simulink model "SF009A_DutyCycThermProtn"  (R2013b)
settings: Solver=FixedStepDiscrete  SolverMode=SingleTasking  StartTime=0.0  StopTime=1  FixedStep=0.1  RelTol=1e-3
values from neighbouring files (symbols this model uses):
  AbsltTThermLimCnt = DataDict.NTC    [SF009A_DutyCycThermProtn_DataDict.m]
  ARCHGLBPRM_100MILLISEC_SEC_F32 = DataDict.Constant    [SF009A_DutyCycThermProtn_DataDict.m]
  CTRLRANDCUTFLT_CNT_U08 = DataDict.Constant    [SF009A_DutyCycThermProtn_DataDict.m]
  CTRLRTFLT_CNT_U08 = DataDict.Constant    [SF009A_DutyCycThermProtn_DataDict.m]
  CUTFLT_CNT_U08 = DataDict.Constant    [SF009A_DutyCycThermProtn_DataDict.m]
  DITHERMLIM_MOTNWTMTR_F32 = DataDict.Constant    [SF009A_DutyCycThermProtn_DataDict.m]
  DutyCycExcddCnt = DataDict.NTC    [SF009A_DutyCycThermProtn_DataDict.m]
  DutyCycThermProtnAbsltCtrlTTblX = DataDict.Calibration    [SF009A_DutyCycThermProtn_DataDict.m]
  DutyCycThermProtnAbsltCtrlTTqTblY = DataDict.Calibration    [SF009A_DutyCycThermProtn_DataDict.m]
  DutyCycThermProtnAbsltCuTTblX = DataDict.Calibration    [SF009A_DutyCycThermProtn_DataDict.m]
  DutyCycThermProtnAbsltCuTTqTblY = DataDict.Calibration    [SF009A_DutyCycThermProtn_DataDict.m]
  DutyCycThermProtnAbsltMotVelBreakPt = DataDict.Calibration    [SF009A_DutyCycThermProtn_DataDict.m]
  DutyCycThermProtnAbsltTTqSlewHiLim = DataDict.Calibration    [SF009A_DutyCycThermProtn_DataDict.m]
  DutyCycThermProtnAbsltTTqSlewLoLim = DataDict.Calibration    [SF009A_DutyCycThermProtn_DataDict.m]
  DutyCycThermProtnCtrlT = DataDict.Calibration    [SF009A_DutyCycThermProtn_DataDict.m]
  DutyCycThermProtnCtrlTSeln = DataDict.Calibration    [SF009A_DutyCycThermProtn_DataDict.m]
  DutyCycThermProtnDutyCycFildThd = DataDict.Calibration    [SF009A_DutyCycThermProtn_DataDict.m]
  DutyCycThermProtnIgnOffCtrlEna = DataDict.Calibration    [SF009A_DutyCycThermProtn_DataDict.m]
  DutyCycThermProtnIgnOffMsgWaitTi = DataDict.Calibration    [SF009A_DutyCycThermProtn_DataDict.m]
  DutyCycThermProtnLstTblValNonStall = DataDict.Calibration    [SF009A_DutyCycThermProtn_DataDict.m]
  DutyCycThermProtnLstTblValStall = DataDict.Calibration    [SF009A_DutyCycThermProtn_DataDict.m]
  DutyCycThermProtnMotPrTSeln = DataDict.Calibration    [SF009A_DutyCycThermProtn_DataDict.m]
  DutyCycThermProtnMplr1NonStallTblY = DataDict.Calibration    [SF009A_DutyCycThermProtn_DataDict.m]
  DutyCycThermProtnMplr1StallTblY = DataDict.Calibration    [SF009A_DutyCycThermProtn_DataDict.m]
  DutyCycThermProtnMplr2NonStallTblY = DataDict.Calibration    [SF009A_DutyCycThermProtn_DataDict.m]
  DutyCycThermProtnMplr2StallTblY = DataDict.Calibration    [SF009A_DutyCycThermProtn_DataDict.m]
  DutyCycThermProtnMplr3NonStallTblY = DataDict.Calibration    [SF009A_DutyCycThermProtn_DataDict.m]
  DutyCycThermProtnMplr3StallTblY = DataDict.Calibration    [SF009A_DutyCycThermProtn_DataDict.m]
  DutyCycThermProtnMplr4NonStallTblY = DataDict.Calibration    [SF009A_DutyCycThermProtn_DataDict.m]
  DutyCycThermProtnMplr4StallTblY = DataDict.Calibration    [SF009A_DutyCycThermProtn_DataDict.m]
  DutyCycThermProtnMplr5NonStallTblY = DataDict.Calibration    [SF009A_DutyCycThermProtn_DataDict.m]
  DutyCycThermProtnMplr5StallTblY = DataDict.Calibration    [SF009A_DutyCycThermProtn_DataDict.m]
  DutyCycThermProtnMplr6NonStallTblY = DataDict.Calibration    [SF009A_DutyCycThermProtn_DataDict.m]
  DutyCycThermProtnMplr6StallTblY = DataDict.Calibration    [SF009A_DutyCycThermProtn_DataDict.m]
  DutyCycThermProtnMplrTblX = DataDict.Calibration    [SF009A_DutyCycThermProtn_DataDict.m]
  DutyCycThermProtnMplrTSeln = DataDict.Calibration    [SF009A_DutyCycThermProtn_DataDict.m]
  DutyCycThermProtnSlowFilTSeln = DataDict.Calibration    [SF009A_DutyCycThermProtn_DataDict.m]
  DutyCycThermProtnThermLimScaFac = DataDict.Calibration    [SF009A_DutyCycThermProtn_DataDict.m]
  DutyCycThermProtnThermLoadLimTblX = DataDict.Calibration    [SF009A_DutyCycThermProtn_DataDict.m]
  DutyCycThermProtnThermLoadLimTblY = DataDict.Calibration    [SF009A_DutyCycThermProtn_DataDict.m]
  DutyCycThermProtnTqCmdSlewDwn = DataDict.Calibration    [SF009A_DutyCycThermProtn_DataDict.m]
  DutyCycThermProtnTqCmdSlewUp = DataDict.Calibration    [SF009A_DutyCycThermProtn_DataDict.m]
  FILVALMIN_ULS_F32 = DataDict.Constant    [SF009A_DutyCycThermProtn_DataDict.m]
  IGNTIOFFTHD_CNT_F32 = DataDict.Constant    [SF009A_DutyCycThermProtn_DataDict.m]
  NODEBSTEP_CNT_U16 = DataDict.Constant    [SF009A_DutyCycThermProtn_DataDict.m]
  ONEPERC_ULS_F32 = DataDict.Constant    [SF009A_DutyCycThermProtn_DataDict.m]
  TAU3_SEC_F32 = DataDict.Constant    [SF009A_DutyCycThermProtn_DataDict.m]
  TAU4_SEC_F32 = DataDict.Constant    [SF009A_DutyCycThermProtn_DataDict.m]
  TAU5_SEC_F32 = DataDict.Constant    [SF009A_DutyCycThermProtn_DataDict.m]
  TAU6_SEC_F32 = DataDict.Constant    [SF009A_DutyCycThermProtn_DataDict.m]
  THERMLOADLIMTBLIDX_ULS_U08 = DataDict.Constant    [SF009A_DutyCycThermProtn_DataDict.m]
undefined symbols (not defined in the file or in its folder): NtcSts1, NvmGetErrSts1
libraries: FixdToFloat x13, Fil x12, NxtrLim x12, simulink x11, NxtrMath x8, FloatToFixd x6, NxtrMax x6, NxtrMin x3, NxtrAbslt x2, NxtrNvM x1
(part 2 of 7)

== system SF009A_DutyCycThermProtn/DutyCycThermProtn/DutyCycThermProtnInit1/NVM_NOK ==
  note: In the event of NVM failure
      | zero out the whole shadow ram image
  Action Port : ActionPort  ActionType=then
  Constant1 : Constant  RequirementInfo={'linktype_rmi_doors' '0000a52a (/E-STEER Core/SubSystem Specifications/Application Functions/SF009A Thermal Duty Cycle Protection)' '#SF009A_285' 'true' 'REQ: SF009A_285' '' } %GIDa_302cae02_0488_4259_b126_8b47f6fdcb2b  Value=0  OutDataTypeStr=Inherit: Inherit via back propagation
  Constant2 : Constant  RequirementInfo={'linktype_rmi_doors' '0000a52a (/E-STEER Core/SubSystem Specifications/Application Functions/SF009A Thermal Duty Cycle Protection)' '#SF009A_285' 'true' 'REQ: SF009A_285' '' } %GIDa_07daeeb8_67fa_455d_b996_6ae10cb4fd0f  Value=0  OutDataTypeStr=Inherit: Inherit via back propagation
  Constant3 : Constant  RequirementInfo={'linktype_rmi_doors' '0000a52a (/E-STEER Core/SubSystem Specifications/Application Functions/SF009A Thermal Duty Cycle Protection)' '#SF009A_285' 'true' 'REQ: SF009A_285' '' } %GIDa_3e650e9f_6932_4571_90f1_f6987a41f5b5  Value=0  OutDataTypeStr=Inherit: Inherit via back propagation
  Constant4 : Constant  RequirementInfo={'linktype_rmi_doors' '0000a52a (/E-STEER Core/SubSystem Specifications/Application Functions/SF009A Thermal Duty Cycle Protection)' '#SF009A_285' 'true' 'REQ: SF009A_285' '' } %GIDa_9674530a_4135_4c18_b828_962e244c35c9  Value=0  OutDataTypeStr=Inherit: Inherit via back propagation
  CopyRight2 : Subsystem  Description=|  mask(Copyright Information){none=on}
      | Copyright info block.                                               
      |                                                                     
      | Place copyright information at the top of every subsystem in design.
      mask prompts: none "No parameters"
      mask help: Place copyright information at the top of every subsystem in design.
      mask Display:
      | NxtrConf = 'Nexteer Confidential';
      | 
      | sys = bdroot; %handle for the current model ("system")
      | first = get_param(sys,'Created');
      | first = first(end-3:end);  %year is last four digits
      | 
      | last = get_param(sys,'LastModifiedDate');
      | if isempty(last)
      |     last = datestr(now,'yyyy');
      | else
      |     last = last(end-3:end);
      | end
      | 
      | if strcmp(first,last)
      |     fprintf('%s -- Copyright %s Nexteer',NxtrConf,first)
      | else
      |     fprintf('%s -- %s%s- %s Nexteer',NxtrConf,char(169),first,last)
      | end
  Data Store Write2 : DataStoreWrite  RequirementInfo={'linktype_rmi_doors' '0000a52a (/E-STEER Core/SubSystem Specifications/Application Functions/SF009A Thermal Duty Cycle Protection)' '#SF009A_285' 'true' 'REQ: SF009A_285' '' } %GIDa_4ceb1b4c_38bc_44b0_9a64_43020f602cc7  Priority=1  DataStoreName=FilStVal  DataStoreElements=FilStVal.Fil3StVal#FilStVal.Fil4StVal#FilStVal.Fil5StVal#FilStVal.Fil6StVal
  wires:
  Constant1/1 -> Data Store Write2/1
  Constant2/1 -> Data Store Write2/2
  Constant4/1 -> Data Store Write2/4
  Constant3/1 -> Data Store Write2/3

== system SF009A_DutyCycThermProtn/DutyCycThermProtn/DutyCycThermProtnInit1/NVM_Ok ==
  Action Port : ActionPort  ActionType=else
  Constant1 : Constant  Value=0  OutDataTypeStr=Inherit: Inherit via back propagation
  CopyRight2 : Subsystem  Description=|  mask(Copyright Information){none=on}
      | Copyright info block.                                               
      |                                                                     
      | Place copyright information at the top of every subsystem in design.
      mask prompts: none "No parameters"
      mask help: Place copyright information at the top of every subsystem in design.
      mask Display:
      | NxtrConf = 'Nexteer Confidential';
      | 
      | sys = bdroot; %handle for the current model ("system")
      | first = get_param(sys,'Created');
      | first = first(end-3:end);  %year is last four digits
      | 
      | last = get_param(sys,'LastModifiedDate');
      | if isempty(last)
      |     last = datestr(now,'yyyy');
      | else
      |     last = last(end-3:end);
      | end
      | 
      | if strcmp(first,last)
      |     fprintf('%s -- Copyright %s Nexteer',NxtrConf,first)
      | else
      |     fprintf('%s -- %s%s- %s Nexteer',NxtrConf,char(169),first,last)
      | end
  Terminator : Terminator
  wires:
  Constant1/1 -> Terminator/1

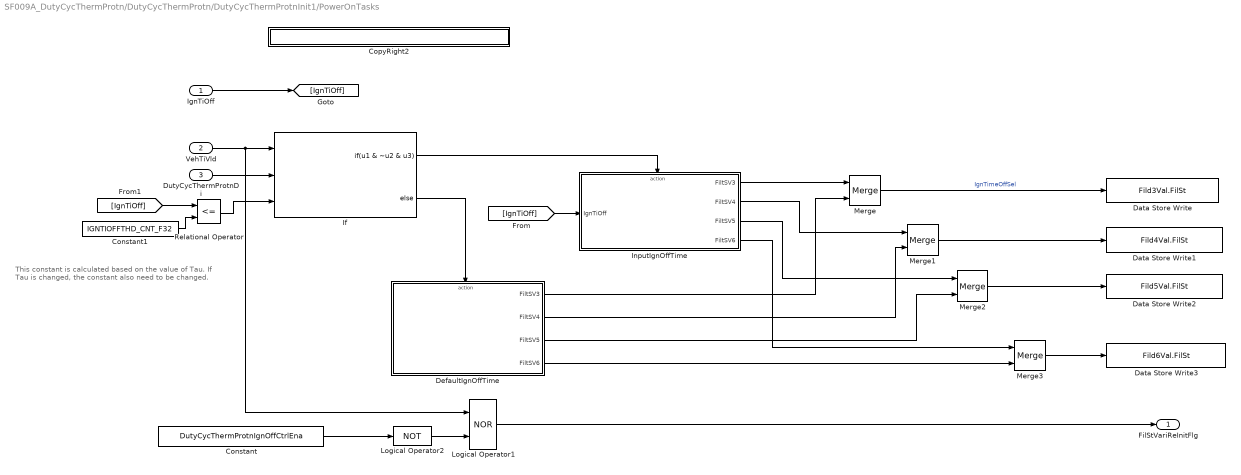
== system SF009A_DutyCycThermProtn/DutyCycThermProtn/DutyCycThermProtnInit1/PowerOnTasks ==
  note: This constant is calculated based on the value of Tau.
      | If Tau is changed, the constant also need to be changed.
  IgnTiOff : Inport
  VehTiVld : Inport  RequirementInfo={'linktype_rmi_doors' '0000a52a (/E-STEER Core/SubSystem Specifications/Application Functions/SF009A Thermal Duty Cycle Protection)' '#SF009A_285' 'true' 'REQ: SF009A_285' '' } %GIDa_9c854dc3_aea9_4b7d_9e72_9615408c52be  Port=2
  DutyCycThermProtnDi : Inport  RequirementInfo={'linktype_rmi_doors' '0000a52a (/E-STEER Core/SubSystem Specifications/Application Functions/SF009A Thermal Duty Cycle Protection)' '#SF009A_285' 'true' 'REQ: SF009A_285' '' } %GIDa_20215133_6a38_4fa5_bfaa_715d5e520197  Port=3
  Constant : Constant  RequirementInfo={'linktype_rmi_doors' '0000a52a (/E-STEER Core/SubSystem Specifications/Application Functions/SF009A Thermal Duty Cycle Protection)' '#SF009A_288' 'true' 'REQ: SF009A_288' '' } %GIDa_d6af1816_8913_46c1_8a5f_e5ae6f6ebd33  Value=DutyCycThermProtnIgnOffCtrlEna
  Constant1 : Constant  RequirementInfo={'linktype_rmi_doors' '0000a52a (/E-STEER Core/SubSystem Specifications/Application Functions/SF009A Thermal Duty Cycle Protection)' '#SF009A_285' 'true' 'REQ: SF009A_285' '' } %GIDa_da13bd96_169e_43ad_9aad_13a1d233c3db  Value=IGNTIOFFTHD_CNT_F32
  CopyRight2 : Subsystem  Description=|  mask(Copyright Information){none=on}
      | Copyright info block.                                               
      |                                                                     
      | Place copyright information at the top of every subsystem in design.
      mask prompts: none "No parameters"
      mask help: Place copyright information at the top of every subsystem in design.
      mask Display:
      | NxtrConf = 'Nexteer Confidential';
      | 
      | sys = bdroot; %handle for the current model ("system")
      | first = get_param(sys,'Created');
      | first = first(end-3:end);  %year is last four digits
      | 
      | last = get_param(sys,'LastModifiedDate');
      | if isempty(last)
      |     last = datestr(now,'yyyy');
      | else
      |     last = last(end-3:end);
      | end
      | 
      | if strcmp(first,last)
      |     fprintf('%s -- Copyright %s Nexteer',NxtrConf,first)
      | else
      |     fprintf('%s -- %s%s- %s Nexteer',NxtrConf,char(169),first,last)
      | end
  Data Store Write : DataStoreWrite  DataStoreName=Fild3Val  DataStoreElements=Fild3Val.FilSt
  Data Store Write1 : DataStoreWrite  DataStoreName=Fild4Val  DataStoreElements=Fild4Val.FilSt
  Data Store Write2 : DataStoreWrite  DataStoreName=Fild5Val  DataStoreElements=Fild5Val.FilSt
  Data Store Write3 : DataStoreWrite  DataStoreName=Fild6Val  DataStoreElements=Fild6Val.FilSt
  DefaultIgnOffTime : Subsystem  RequirementInfo={} %GIDa_e2463be5_64da_4144_9cc6_dd109eab91a1  TreatAsAtomicUnit=on
  If : If  RequirementInfo={'linktype_rmi_doors' '0000a52a (/E-STEER Core/SubSystem Specifications/Application Functions/SF009A Thermal Duty Cycle Protection)' '#SF009A_285' 'true' 'REQ: SF009A_285' '' } %GIDa_3e38b5b9_0c5d_47ab_89b1_64e918870a53  NumInputs=3  IfExpression=u1 & ~u2 & u3
  InputIgnOffTime : Subsystem  RequirementInfo={} %GIDa_43daa1c3_65fe_4cdd_94a1_b7322396a1ac  TreatAsAtomicUnit=on
  Logical Operator1 : Logic  RequirementInfo={'linktype_rmi_doors' '0000a52a (/E-STEER Core/SubSystem Specifications/Application Functions/SF009A Thermal Duty Cycle Protection)' '#SF009A_280' 'true' 'REQ: SF009A_280' '' } %GIDa_edbebf0e_bcf8_4967_a510_970fba2b2e0b  Operator=NOR  AllPortsSameDT=off  OutDataTypeStr=boolean
  Logical Operator2 : Logic  RequirementInfo={'linktype_rmi_doors' '0000a52a (/E-STEER Core/SubSystem Specifications/Application Functions/SF009A Thermal Duty Cycle Protection)' '#SF009A_280' 'true' 'REQ: SF009A_280' '' } %GIDa_f304b822_166f_4701_8c8b_94ad225b72e6  Operator=NOT  AllPortsSameDT=off  OutDataTypeStr=boolean
  Merge : Merge  RequirementInfo={} %GIDa_1e03ac42_f159_46b0_a200_7b6c92e2721c
  Merge1 : Merge  RequirementInfo={} %GIDa_32e162cf_165c_4a40_9f13_19e0e5e6e227
  Merge2 : Merge  RequirementInfo={} %GIDa_493fd6f9_28e3_4a2f_8c16_2836a030636e
  Merge3 : Merge  RequirementInfo={} %GIDa_b95078aa_c4af_4ddb_8213_bc830cf1fee0
  Relational Operator : RelationalOperator  RequirementInfo={'linktype_rmi_doors' '0000a52a (/E-STEER Core/SubSystem Specifications/Application Functions/SF009A Thermal Duty Cycle Protection)' '#SF009A_285' 'true' 'REQ: SF009A_285' '' } %GIDa_8a99ca10_b364_4588_b658_259f4470d472  Operator=<=  OutDataTypeStr=boolean
  FilStVariReInitFlg : Outport
  wires:
  Logical Operator1/1 -> FilStVariReInitFlg/1
  Constant/1 -> Logical Operator2/1
  VehTiVld/1 -> If/1, Logical Operator1/1
  Logical Operator2/1 -> Logical Operator1/2
  DutyCycThermProtnDi/1 -> If/2
  [IgnTiOff] -> InputIgnOffTime/1(IgnTiOff)
  If/1 -> InputIgnOffTime/Action
  InputIgnOffTime/1(FiltSV3) -> Merge/1
  DefaultIgnOffTime/1(FiltSV3) -> Merge/2
  If/2 -> DefaultIgnOffTime/Action
  IgnTiOff/1 -> [IgnTiOff]
  [IgnTiOff] -> Relational Operator/1
  Constant1/1 -> Relational Operator/2
  Relational Operator/1 -> If/3
  DefaultIgnOffTime/2(FiltSV4) -> Merge1/2
  InputIgnOffTime/2(FiltSV4) -> Merge1/1
  InputIgnOffTime/3(FiltSV5) -> Merge2/1
  DefaultIgnOffTime/3(FiltSV5) -> Merge2/2
  InputIgnOffTime/4(FiltSV6) -> Merge3/1
  DefaultIgnOffTime/4(FiltSV6) -> Merge3/2
  Merge3/1 -> Data Store Write3/1
  Merge2/1 -> Data Store Write2/1
  Merge1/1 -> Data Store Write1/1
  Merge/1 -> Data Store Write/1  "IgnTimeOffSel"

== system SF009A_DutyCycThermProtn/DutyCycThermProtn/DutyCycThermProtnInit1/SetInitialValueOfAbsTempLimitSlew ==
  note: This subsystem sets the initial value of the "AbsltTLimSlewStVari"
      | which is used as state variable of rate limiter block in Per1 subsystem.
  Constant2 : Constant  Value=0
  Copyright1 : Subsystem  Description=|  RequirementInfo={} %GIDa_1a6fa9aa_8716_46b8_8e70_044847d882f9  mask(Copyright Information){none=on}
      | Copyright info block.                                               
      |                                                                     
      | Place copyright information at the top of every subsystem in design.
      mask prompts: none "No parameters"
      mask help: Place copyright information at the top of every subsystem in design.
      mask Display:
      | NxtrConf = 'Nexteer Confidential';
      | 
      | sys = bdroot; %handle for the current model ("system")
      | first = get_param(sys,'Created');
      | if(isempty(first))
      |     first = datestr(now,'yyyy');
      | else
      |     first = first(end-3:end);  %year is last four digits
      | end
      | 
      | last = get_param(sys,'LastModifiedDate');
      | if isempty(last)
      |     last = datestr(now,'yyyy');
      | else
      |     last = last(end-3:end);
      | end
      | 
      | if strcmp(first,last)
      |     fprintf('%s\nCopyright  %s Nexteer',NxtrConf,first);
      | else
      |     fprintf('%s\n%s%s-%s Nexteer',NxtrConf,char(169),first,last);
      | end
  Data Store Write : DataStoreWrite  DataStoreName=AbsltTLimSlewStVari
  FixdToFloat_f32_u16 : FixdToFloat/FixdToFloat_f32_u16  Param1=7
  Selector2 : Selector  IndexMode=Zero-based  InputPortWidth=4  IndexOptions=Index vector (port)  Indices=[1 3]  OutputSizes=1
  const2 : Constant  Value=DutyCycThermProtnAbsltCtrlTTqTblY
  wires:
  Selector2/1 -> FixdToFloat_f32_u16/1
  const2/1 -> Selector2/1
  Constant2/1 -> Selector2/2
  FixdToFloat_f32_u16/1 -> Data Store Write/1

== system SF009A_DutyCycThermProtn/DutyCycThermProtn/DutyCycThermProtnInit1/SetInitialValueOfLstTblValRateLimrStVari ==
  note: Last value of the table "DutyCycThermProtnThermLoadLimTblY" is selected and assigned to "LstTblValRateLimrStVari".
  note: This subsystem sets the initial value of the "LstTblValRateLimrStVari"
      | which is used as state variable of rate limiter block in Per1 subsystem.
  Add : Sum  Inputs=+-
  Constant1 : Constant  OutDataTypeStr=uint8
  Constant3 : Constant  Value=THERMLOADLIMTBLIDX_ULS_U08
  Copyright1 : Subsystem  Description=|  RequirementInfo={} %GIDa_56626e63_5a4b_4b9f_b0a2_c0ad22b87c06  mask(Copyright Information){none=on}
      | Copyright info block.                                               
      |                                                                     
      | Place copyright information at the top of every subsystem in design.
      mask prompts: none "No parameters"
      mask help: Place copyright information at the top of every subsystem in design.
      mask Display:
      | NxtrConf = 'Nexteer Confidential';
      | 
      | sys = bdroot; %handle for the current model ("system")
      | first = get_param(sys,'Created');
      | if(isempty(first))
      |     first = datestr(now,'yyyy');
      | else
      |     first = first(end-3:end);  %year is last four digits
      | end
      | 
      | last = get_param(sys,'LastModifiedDate');
      | if isempty(last)
      |     last = datestr(now,'yyyy');
      | else
      |     last = last(end-3:end);
      | end
      | 
      | if strcmp(first,last)
      |     fprintf('%s\nCopyright  %s Nexteer',NxtrConf,first);
      | else
      |     fprintf('%s\n%s%s-%s Nexteer',NxtrConf,char(169),first,last);
      | end
  Data Store Write : DataStoreWrite  DataStoreName=LstTblValRateLimrStVari
  FixdToFloat_f32_u16 : FixdToFloat/FixdToFloat_f32_u16  Param1=7
  Selector2 : Selector  IndexMode=Zero-based  InputPortWidth=8  IndexOptions=Index vector (port)  Indices=[1 3]  OutputSizes=1
  const1 : Constant  Value=DutyCycThermProtnThermLoadLimTblY
  wires:
  const1/1 -> Selector2/1
  Constant3/1 -> Add/1
  FixdToFloat_f32_u16/1 -> Data Store Write/1
  Selector2/1 -> FixdToFloat_f32_u16/1
  Constant1/1 -> Add/2
  Add/1 -> Selector2/2

== system SF009A_DutyCycThermProtn/DutyCycThermProtn/DutyCycThermProtnPer1/CopyRight2 ==

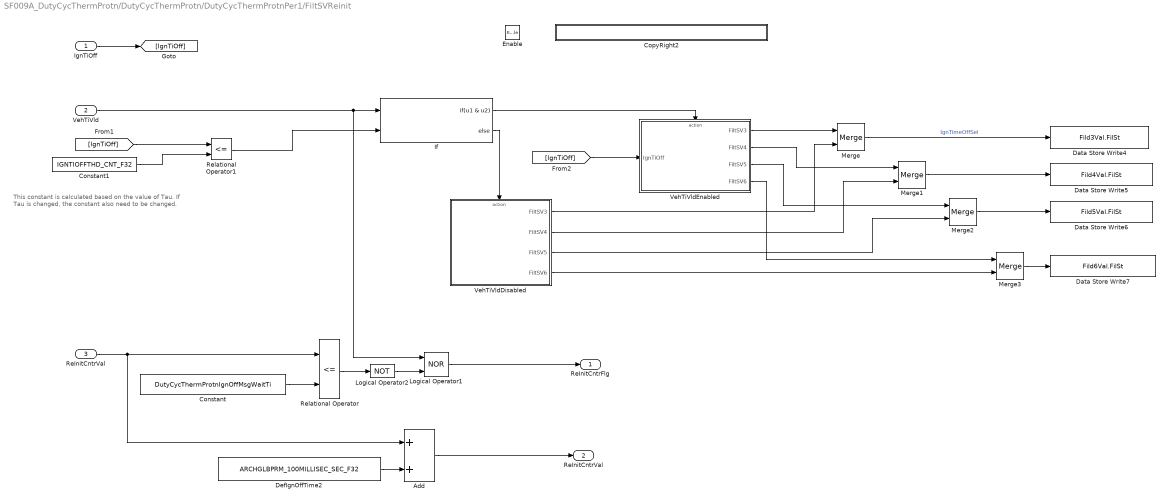
== system SF009A_DutyCycThermProtn/DutyCycThermProtn/DutyCycThermProtnPer1/FiltSVReinit ==
  note: This constant is calculated based on the value of Tau.
      | If Tau is changed, the constant also need to be changed.
  "IgnTiOff " : Inport
  VehTiVld : Inport  RequirementInfo={'linktype_rmi_doors' '0000a52a (/E-STEER Core/SubSystem Specifications/Application Functions/SF009A Thermal Duty Cycle Protection)' '#SF009A_285' 'true' 'REQ: SF009A_285' '' } %GIDa_f2cd1e6f_4c09_4c7d_bb23_8c8b610d12b5  Port=2
  "ReInitCntrVal " : Inport  Port=3
  Enable : EnablePort
  Add : Sum  RequirementInfo={'linktype_rmi_doors' '0000a52a (/E-STEER Core/SubSystem Specifications/Application Functions/SF009A Thermal Duty Cycle Protection)' '#SF009A_280' 'true' 'REQ: SF009A_280' '' } %GIDa_580a5325_9da3_4dde_9987_9ed8cd772d3d
  Constant : Constant  RequirementInfo={'linktype_rmi_doors' '0000a52a (/E-STEER Core/SubSystem Specifications/Application Functions/SF009A Thermal Duty Cycle Protection)' '#SF009A_280' 'true' 'REQ: SF009A_280' '' } %GIDa_c76ac90e_c62d_4456_ae2a_df3b21a2a4e0  Value=DutyCycThermProtnIgnOffMsgWaitTi
  Constant1 : Constant  RequirementInfo={'linktype_rmi_doors' '0000a52a (/E-STEER Core/SubSystem Specifications/Application Functions/SF009A Thermal Duty Cycle Protection)' '#SF009A_285' 'true' 'REQ: SF009A_285' '' } %GIDa_846e87e9_58bc_4580_b93b_af0c098bc72a  Value=IGNTIOFFTHD_CNT_F32
  CopyRight2 : Subsystem  Description=|  mask(Copyright Information){none=on}
      | Copyright info block.                                               
      |                                                                     
      | Place copyright information at the top of every subsystem in design.
      mask prompts: none "No parameters"
      mask help: Place copyright information at the top of every subsystem in design.
      mask Display:
      | NxtrConf = 'Nexteer Confidential';
      | 
      | sys = bdroot; %handle for the current model ("system")
      | first = get_param(sys,'Created');
      | first = first(end-3:end);  %year is last four digits
      | 
      | last = get_param(sys,'LastModifiedDate');
      | if isempty(last)
      |     last = datestr(now,'yyyy');
      | else
      |     last = last(end-3:end);
      | end
      | 
      | if strcmp(first,last)
      |     fprintf('%s -- Copyright %s Nexteer',NxtrConf,first)
      | else
      |     fprintf('%s -- %s%s- %s Nexteer',NxtrConf,char(169),first,last)
      | end
  Data Store Write4 : DataStoreWrite  DataStoreName=Fild3Val  DataStoreElements=Fild3Val.FilSt
  Data Store Write5 : DataStoreWrite  DataStoreName=Fild4Val  DataStoreElements=Fild4Val.FilSt
  Data Store Write6 : DataStoreWrite  DataStoreName=Fild5Val  DataStoreElements=Fild5Val.FilSt
  Data Store Write7 : DataStoreWrite  DataStoreName=Fild6Val  DataStoreElements=Fild6Val.FilSt
  DefIgnOffTime2 : Constant  RequirementInfo={'linktype_rmi_doors' '0000a52a (/E-STEER Core/SubSystem Specifications/Application Functions/SF009A Thermal Duty Cycle Protection)' '#SF009A_280' 'true' 'REQ: SF009A_280' '' } %GIDa_5fa57ba4_c528_4fb6_a79f_ab3413b38764  Value=ARCHGLBPRM_100MILLISEC_SEC_F32
  If : If  RequirementInfo={'linktype_rmi_doors' '0000a52a (/E-STEER Core/SubSystem Specifications/Application Functions/SF009A Thermal Duty Cycle Protection)' '#SF009A_285' 'true' 'REQ: SF009A_285' '' } %GIDa_6e003379_c095_4539_a389_1aacbace0d02  NumInputs=2  IfExpression=u1 & u2
  Logical Operator1 : Logic  RequirementInfo={'linktype_rmi_doors' '0000a52a (/E-STEER Core/SubSystem Specifications/Application Functions/SF009A Thermal Duty Cycle Protection)' '#SF009A_280' 'true' 'REQ: SF009A_280' '' } %GIDa_284f8ad3_0460_4306_9723_53fb8582929e  Operator=NOR  AllPortsSameDT=off  OutDataTypeStr=boolean
  Logical Operator2 : Logic  RequirementInfo={'linktype_rmi_doors' '0000a52a (/E-STEER Core/SubSystem Specifications/Application Functions/SF009A Thermal Duty Cycle Protection)' '#SF009A_280' 'true' 'REQ: SF009A_280' '' } %GIDa_ec00b3f8_66ee_40a8_b7f7_19a445abbf83  Operator=NOT  AllPortsSameDT=off  OutDataTypeStr=boolean
  Merge : Merge  RequirementInfo={} %GIDa_fbbdd3d2_97f2_48a8_a46c_7182b36b6720
  Merge1 : Merge  RequirementInfo={} %GIDa_e9f01da1_ad1a_48a2_b9b1_8b84a4874e09
  Merge2 : Merge  RequirementInfo={} %GIDa_ac698b32_b42d_493c_a1a9_4f85f963d138
  Merge3 : Merge  RequirementInfo={} %GIDa_ea067629_621b_4d75_9cda_f744346af075
  Relational Operator : RelationalOperator  RequirementInfo={'linktype_rmi_doors' '0000a52a (/E-STEER Core/SubSystem Specifications/Application Functions/SF009A Thermal Duty Cycle Protection)' '#SF009A_280' 'true' 'REQ: SF009A_280' '' } %GIDa_3f2901e1_9a76_40d7_87e1_0b54f413400c  Operator=<=  OutDataTypeStr=boolean
  Relational Operator1 : RelationalOperator  RequirementInfo={'linktype_rmi_doors' '0000a52a (/E-STEER Core/SubSystem Specifications/Application Functions/SF009A Thermal Duty Cycle Protection)' '#SF009A_285' 'true' 'REQ: SF009A_285' '' } %GIDa_8f6b1d28_5bfc_46ec_8742_0f7436e122d1  Operator=<=  OutDataTypeStr=boolean
  VehTiVldDisabled : Subsystem  RequirementInfo={} %GIDa_324970fa_b22f_49af_a8a8_20d743678a1e  TreatAsAtomicUnit=on
  VehTiVldEnabled : Subsystem  RequirementInfo={} %GIDa_999d4a90_5417_41b8_9c74_fb77c55787e8  TreatAsAtomicUnit=on
  ReInitCntrFlg : Outport
  ReInitCntrVal : Outport  Port=2
  wires:
  VehTiVld/1 -> Logical Operator1/1, If/1
  Relational Operator/1 -> Logical Operator2/1
  Logical Operator1/1 -> ReInitCntrFlg/1
  Constant/1 -> Relational Operator/2
  "ReInitCntrVal "/1 -> Relational Operator/1, Add/1
  DefIgnOffTime2/1 -> Add/2
  Add/1 -> ReInitCntrVal/1
  Logical Operator2/1 -> Logical Operator1/2
  "IgnTiOff "/1 -> [IgnTiOff]
  If/1 -> VehTiVldEnabled/Action
  If/2 -> VehTiVldDisabled/Action
  VehTiVldEnabled/1(FiltSV3) -> Merge/1
  VehTiVldDisabled/1(FiltSV3) -> Merge/2
  VehTiVldEnabled/2(FiltSV4) -> Merge1/1
  VehTiVldDisabled/2(FiltSV4) -> Merge1/2
  VehTiVldEnabled/3(FiltSV5) -> Merge2/1
  VehTiVldDisabled/3(FiltSV5) -> Merge2/2
  VehTiVldDisabled/4(FiltSV6) -> Merge3/2
  VehTiVldEnabled/4(FiltSV6) -> Merge3/1
  Merge/1 -> Data Store Write4/1  "IgnTimeOffSel"
  Merge1/1 -> Data Store Write5/1
  Merge2/1 -> Data Store Write6/1
  Merge3/1 -> Data Store Write7/1
  Constant1/1 -> Relational Operator1/2
  [IgnTiOff] -> Relational Operator1/1
  Relational Operator1/1 -> If/2
  [IgnTiOff] -> VehTiVldEnabled/1(IgnTiOff)

== system SF009A_DutyCycThermProtn/DutyCycThermProtn/DutyCycThermProtnPer1/LoadLimiting ==
  MotCurrPeakEstimd : Inport
  MotCurrPeakEstimdFild : Inport  Port=2
  MotVelCrf : Inport  Port=3
  Mult12Temp : Inport  Port=4
  Mult36Temp : Inport  Port=5
  SlcTemp : Inport  Port=6
  DutyCycThermProtnDi : Inport  Port=7
  CopyRight2 : Subsystem  Description=|  mask(Copyright Information){none=on}
      | Copyright info block.                                               
      |                                                                     
      | Place copyright information at the top of every subsystem in design.
      mask prompts: none "No parameters"
      mask help: Place copyright information at the top of every subsystem in design.
      mask Display:
      | NxtrConf = 'Nexteer Confidential';
      | 
      | sys = bdroot; %handle for the current model ("system")
      | first = get_param(sys,'Created');
      | first = first(end-3:end);  %year is last four digits
      | 
      | last = get_param(sys,'LastModifiedDate');
      | if isempty(last)
      |     last = datestr(now,'yyyy');
      | else
      |     last = last(end-3:end);
      | end
      | 
      | if strcmp(first,last)
      |     fprintf('%s -- Copyright %s Nexteer',NxtrConf,first)
      | else
      |     fprintf('%s -- %s%s- %s Nexteer',NxtrConf,char(169),first,last)
      | end
  FilterPercMax : Subsystem  RequirementInfo={'linktype_rmi_doors' '0000a52a (/E-STEER Core/SubSystem Specifications/Application Functions/SF009A Thermal Duty Cycle Protection)' '#SF009A_117' 'true' 'REQ: SF009A_117' '' ; 'linktype_rmi_doors' '0000a52a (/E-STEER Core/SubSystem Specifications/Application Functions/SF009A Thermal Duty Cycle Protection)' '#SF009A_164' 'true' 'REQ: SF009A_164' '' ; 'linktype_rmi_doors' '0000a52a (/E-STEER Core/SubSystem Specifications/Application Functions/SF009A Thermal Duty Cycle Protection)' '#SF009A_167' 'true' 'REQ: SF009A_167' '' } %GIDa_3ed6a9be_a9c0_4455_85d8_2437f2a07ac3
  Multiplier : Subsystem  RequirementInfo={'linktype_rmi_doors' '0000a52a (/E-STEER Core/SubSystem Specifications/Application Functions/SF009A Thermal Duty Cycle Protection)' '#SF009A_155' 'true' 'REQ: SF009A_155' '' } %GIDa_6617263c_fa09_4775_af12_9c4ea5a67b95
  PowerOffTasks : Subsystem  RequirementInfo={} %GIDa_972c5a1a_4225_44ec_a602_2278b884c0a1
  ThermalLoadLimit : Subsystem  RequirementInfo={} %GIDa_b466cb19_a628_4d86_8b51_80f6cd1be6a8
  ThermLimSlowFilMax : Outport
  DutyCycThermProtnMaxOutp : Outport  Port=2
  ThermalLoadLmt : Outport  Port=3
  wires:
  Mult12Temp/1 -> Multiplier/1(Mult12Temp)
  Mult36Temp/1 -> Multiplier/2(Mult36Temp)
  MotCurrPeakEstimd/1 -> FilterPercMax/7(MotCurrPeakEstimd)
  MotCurrPeakEstimdFild/1 -> FilterPercMax/8(MotCurrPeakEstimdFild)
  ThermalLoadLimit/1(ThermalLoadLmt) -> ThermalLoadLmt/1
  FilterPercMax/1(MaxOut) -> ThermalLoadLimit/3(MaxOut), DutyCycThermProtnMaxOutp/1
  SlcTemp/1 -> ThermalLoadLimit/2(SlcTemp)
  FilterPercMax/2(ThermLimSlowFilMax) -> ThermLimSlowFilMax/1
  Multiplier/1(Mult1) -> FilterPercMax/1(Mult1)
  Multiplier/2(Mult2) -> FilterPercMax/2(Mult2)
  Multiplier/3(Mult3) -> FilterPercMax/3(Mult3)
  Multiplier/4(Mult4) -> FilterPercMax/4(Mult4)
  Multiplier/5(Mult5) -> FilterPercMax/5(Mult5)
  Multiplier/6(Mult6) -> FilterPercMax/6(Mult6)
  MotVelCrf/1 -> Multiplier/3(MotVelCrf), [MtrVel]
  [MtrVel] -> ThermalLoadLimit/1(MotVelCrf)
  DutyCycThermProtnDi/1 -> FilterPercMax/9(DutyCycThermProtnDi)

== system SF009A_DutyCycThermProtn/DutyCycThermProtn/DutyCycThermProtnPer1/ServiceDefeatFiltSVReinit ==
  Enable : EnablePort
  CopyRight2 : Subsystem  Description=|  mask(Copyright Information){none=on}
      | Copyright info block.                                               
      |                                                                     
      | Place copyright information at the top of every subsystem in design.
      mask prompts: none "No parameters"
      mask help: Place copyright information at the top of every subsystem in design.
      mask Display:
      | NxtrConf = 'Nexteer Confidential';
      | 
      | sys = bdroot; %handle for the current model ("system")
      | first = get_param(sys,'Created');
      | first = first(end-3:end);  %year is last four digits
      | 
      | last = get_param(sys,'LastModifiedDate');
      | if isempty(last)
      |     last = datestr(now,'yyyy');
      | else
      |     last = last(end-3:end);
      | end
      | 
      | if strcmp(first,last)
      |     fprintf('%s -- Copyright %s Nexteer',NxtrConf,first)
      | else
      |     fprintf('%s -- %s%s- %s Nexteer',NxtrConf,char(169),first,last)
      | end
  Data Store Write : DataStoreWrite  DataStoreName=Fild3Val  DataStoreElements=Fild3Val.FilSt
  Data Store Write1 : DataStoreWrite  DataStoreName=Fild4Val  DataStoreElements=Fild4Val.FilSt
  Data Store Write2 : DataStoreWrite  DataStoreName=Fild5Val  DataStoreElements=Fild5Val.FilSt
  Data Store Write3 : DataStoreWrite  DataStoreName=Fild6Val  DataStoreElements=Fild6Val.FilSt
  DefIgnOffTime1 : Constant  Value=FILVALMIN_ULS_F32
  wires:
  DefIgnOffTime1/1 -> Data Store Write2/1, Data Store Write3/1, Data Store Write1/1, Data Store Write/1

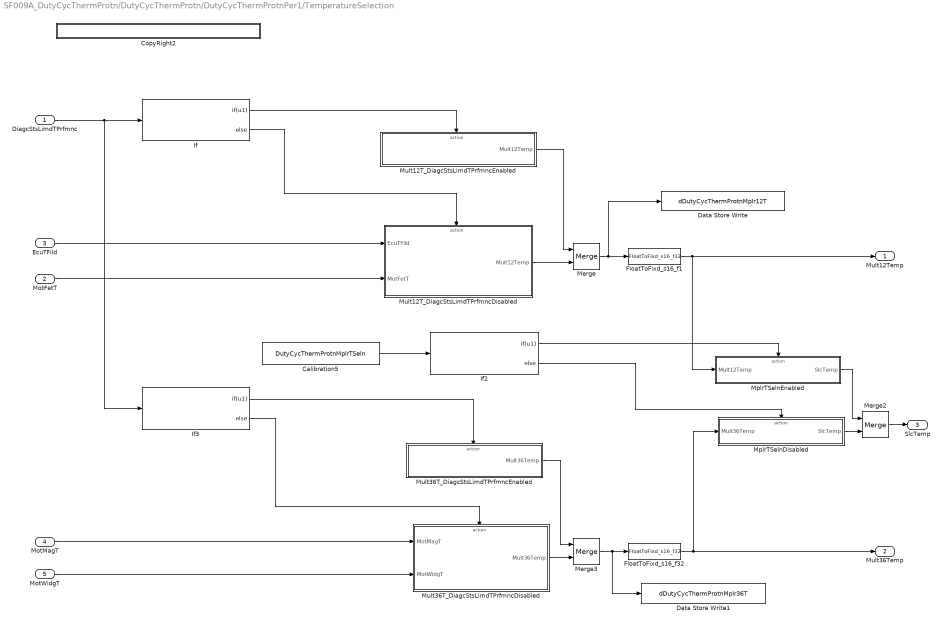
== system SF009A_DutyCycThermProtn/DutyCycThermProtn/DutyCycThermProtnPer1/TemperatureSelection ==
  DiagcStsLimdTPrfmnc : Inport
  MotFetT : Inport  Port=2
  EcuTFild : Inport  Port=3
  MotMagT : Inport  Port=4
  MotWidgT : Inport  Port=5
  Calibration5 : Constant  RequirementInfo={'linktype_rmi_doors' '0000a52a (/E-STEER Core/SubSystem Specifications/Application Functions/SF009A Thermal Duty Cycle Protection)' '#SF009A_114' 'true' 'REQ: SF009A_114' '' } %GIDa_8e23093e_27f7_4ecb_a00e_278a1ac33baa  Value=DutyCycThermProtnMplrTSeln
  CopyRight2 : Subsystem  Description=|  mask(Copyright Information){none=on}
      | Copyright info block.                                               
      |                                                                     
      | Place copyright information at the top of every subsystem in design.
      mask prompts: none "No parameters"
      mask help: Place copyright information at the top of every subsystem in design.
      mask Display:
      | NxtrConf = 'Nexteer Confidential';
      | 
      | sys = bdroot; %handle for the current model ("system")
      | first = get_param(sys,'Created');
      | first = first(end-3:end);  %year is last four digits
      | 
      | last = get_param(sys,'LastModifiedDate');
      | if isempty(last)
      |     last = datestr(now,'yyyy');
      | else
      |     last = last(end-3:end);
      | end
      | 
      | if strcmp(first,last)
      |     fprintf('%s -- Copyright %s Nexteer',NxtrConf,first)
      | else
      |     fprintf('%s -- %s%s- %s Nexteer',NxtrConf,char(169),first,last)
      | end
  Data Store Write : DataStoreWrite  DataStoreName=dDutyCycThermProtnMplr12T
  Data Store Write1 : DataStoreWrite  DataStoreName=dDutyCycThermProtnMplr36T
  FloatToFixd_s16_f1 : FloatToFixd/FloatToFixd_s16_f32  Param1=0
  FloatToFixd_s16_f32 : FloatToFixd/FloatToFixd_s16_f32  Param1=0
  If : If  RequirementInfo={'linktype_rmi_doors' '0000a52a (/E-STEER Core/SubSystem Specifications/Application Functions/SF009A Thermal Duty Cycle Protection)' '#SF009A_184' 'true' 'REQ: SF009A_184' '' } %GIDa_ca8a8c74_c39c_4f29_8ea9_80465840cae0  IfExpression=u1
  If2 : If  RequirementInfo={'linktype_rmi_doors' '0000a52a (/E-STEER Core/SubSystem Specifications/Application Functions/SF009A Thermal Duty Cycle Protection)' '#SF009A_114' 'true' 'REQ: SF009A_114' '' } %GIDa_9b47838e_1e46_4d53_a4ac_947f8f2c2970  IfExpression=u1
  If3 : If  RequirementInfo={'linktype_rmi_doors' '0000a52a (/E-STEER Core/SubSystem Specifications/Application Functions/SF009A Thermal Duty Cycle Protection)' '#SF009A_188' 'true' 'REQ: SF009A_188' '' } %GIDa_e0f30479_aede_45c0_8abe_02078f308a8d  IfExpression=u1
  Merge : Merge  RequirementInfo={'linktype_rmi_doors' '0000a52a (/E-STEER Core/SubSystem Specifications/Application Functions/SF009A Thermal Duty Cycle Protection)' '#SF009A_184' 'true' 'REQ: SF009A_184' '' } %GIDa_1e2f67ed_7672_410c_a92f_4fda9fc6bd3d
  Merge2 : Merge  RequirementInfo={'linktype_rmi_doors' '0000a52a (/E-STEER Core/SubSystem Specifications/Application Functions/SF009A Thermal Duty Cycle Protection)' '#SF009A_114' 'true' 'REQ: SF009A_114' '' } %GIDa_8d348bab_bea0_492a_9b59_59bbd08be9d5
  Merge3 : Merge  RequirementInfo={'linktype_rmi_doors' '0000a52a (/E-STEER Core/SubSystem Specifications/Application Functions/SF009A Thermal Duty Cycle Protection)' '#SF009A_188' 'true' 'REQ: SF009A_188' '' } %GIDa_5df8e3ee_3e2f_4cf5_813e_794d96b1672c
  MplrTSelnDisabled : Subsystem  RequirementInfo={'linktype_rmi_doors' '0000a52a (/E-STEER Core/SubSystem Specifications/Application Functions/SF009A Thermal Duty Cycle Protection)' '#SF009A_114' 'true' 'REQ: SF009A_114' '' } %GIDa_152d6577_ddba_4ed6_964d_7fee3b02f844  TreatAsAtomicUnit=on
  MplrTSelnEnabled : Subsystem  RequirementInfo={'linktype_rmi_doors' '0000a52a (/E-STEER Core/SubSystem Specifications/Application Functions/SF009A Thermal Duty Cycle Protection)' '#SF009A_114' 'true' 'REQ: SF009A_114' '' } %GIDa_cce2fbea_6a9c_432f_a513_853a7592208d  TreatAsAtomicUnit=on
  Mult12T_DiagcStsLimdTPrfmncDisabled : Subsystem  RequirementInfo={'linktype_rmi_doors' '0000a52a (/E-STEER Core/SubSystem Specifications/Application Functions/SF009A Thermal Duty Cycle Protection)' '#SF009A_184' 'true' 'REQ: SF009A_184' '' ; 'linktype_rmi_doors' '0000a52a (/E-STEER Core/SubSystem Specifications/Application Functions/SF009A Thermal Duty Cycle Protection)' '#SF009A_113' 'true' 'REQ: SF009A_113' '' } %GIDa_200d0c66_213e_4297_a369_dd30af9723bb  TreatAsAtomicUnit=on
  Mult12T_DiagcStsLimdTPrfmncEnabled : Subsystem  RequirementInfo={'linktype_rmi_doors' '0000a52a (/E-STEER Core/SubSystem Specifications/Application Functions/SF009A Thermal Duty Cycle Protection)' '#SF009A_184' 'true' 'REQ: SF009A_184' '' } %GIDa_a9e4a746_b9d3_4349_8af5_fb55dffcf03f  TreatAsAtomicUnit=on
  Mult36T_DiagcStsLimdTPrfmncDisabled : Subsystem  RequirementInfo={'linktype_rmi_doors' '0000a52a (/E-STEER Core/SubSystem Specifications/Application Functions/SF009A Thermal Duty Cycle Protection)' '#SF009A_188' 'true' 'REQ: SF009A_188' '' } %GIDa_17a2b618_a048_49df_aed6_3d93cb514db0  TreatAsAtomicUnit=on
  Mult36T_DiagcStsLimdTPrfmncEnabled : Subsystem  RequirementInfo={'linktype_rmi_doors' '0000a52a (/E-STEER Core/SubSystem Specifications/Application Functions/SF009A Thermal Duty Cycle Protection)' '#SF009A_188' 'true' 'REQ: SF009A_188' '' } %GIDa_4fbf05a2_f454_40fb_8004_56fda0debb36  TreatAsAtomicUnit=on
  Mult12Temp : Outport
  Mult36Temp : Outport  Port=2
  SlcTemp : Outport  Port=3
  wires:
  Mult12T_DiagcStsLimdTPrfmncEnabled/1(Mult12Temp) -> Merge/1
  Mult12T_DiagcStsLimdTPrfmncDisabled/1(Mult12Temp) -> Merge/2
  MplrTSelnEnabled/1(SlcTemp) -> Merge2/1
  MplrTSelnDisabled/1(SlcTemp) -> Merge2/2
  Mult36T_DiagcStsLimdTPrfmncEnabled/1(Mult36Temp) -> Merge3/1
  Mult36T_DiagcStsLimdTPrfmncDisabled/1(Mult36Temp) -> Merge3/2
  DiagcStsLimdTPrfmnc/1 -> If3/1, If/1
  Calibration5/1 -> If2/1
  Merge/1 -> FloatToFixd_s16_f1/1, Data Store Write/1
  Merge3/1 -> FloatToFixd_s16_f32/1, Data Store Write1/1
  Merge2/1 -> SlcTemp/1
  If/1 -> Mult12T_DiagcStsLimdTPrfmncEnabled/Action
  If/2 -> Mult12T_DiagcStsLimdTPrfmncDisabled/Action
  If3/1 -> Mult36T_DiagcStsLimdTPrfmncEnabled/Action
  If3/2 -> Mult36T_DiagcStsLimdTPrfmncDisabled/Action
  If2/1 -> MplrTSelnEnabled/Action
  If2/2 -> MplrTSelnDisabled/Action
  MotFetT/1 -> Mult12T_DiagcStsLimdTPrfmncDisabled/2(MotFetT)
  EcuTFild/1 -> Mult12T_DiagcStsLimdTPrfmncDisabled/1(EcuTFild)
  MotMagT/1 -> Mult36T_DiagcStsLimdTPrfmncDisabled/1(MotMagT)
  MotWidgT/1 -> Mult36T_DiagcStsLimdTPrfmncDisabled/2(MotWidgT)
  FloatToFixd_s16_f32/1 -> Mult36Temp/1, MplrTSelnDisabled/1(Mult36Temp)
  FloatToFixd_s16_f1/1 -> Mult12Temp/1, MplrTSelnEnabled/1(Mult12Temp)

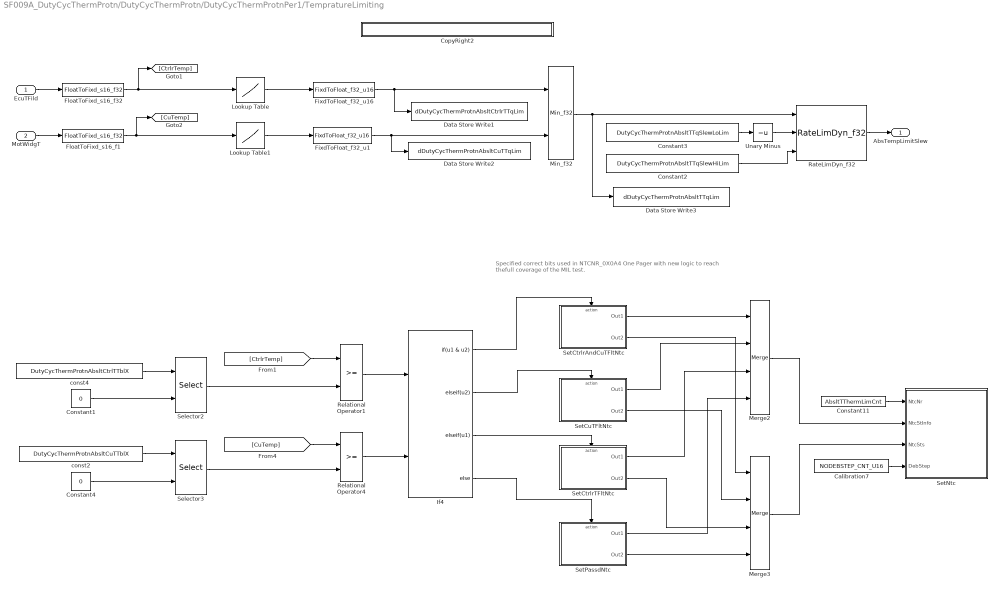
== system SF009A_DutyCycThermProtn/DutyCycThermProtn/DutyCycThermProtnPer1/TempratureLimiting ==
  note: Specified correct bits used in NTCNR_0X0A4 One Pager with new logic to
      |   reach thefull coverage of the MIL test.
  EcuTFild : Inport
  MotWidgT : Inport  Port=2
  Calibration7 : Constant  RequirementInfo={} %GIDa_29bc1e14_3b46_4c24_b28a_4219c883deca  Value=NODEBSTEP_CNT_U16
  Constant1 : Constant  RequirementInfo={'linktype_rmi_doors' '0000a52a (/E-STEER Core/SubSystem Specifications/Application Functions/SF009A Thermal Duty Cycle Protection)' '#SF009A_248' 'true' 'REQ: SF009A_248' '' } %GIDa_58140072_2bca_4ee8_a288_e32bd462a4b4  Value=0
  Constant11 : Constant  RequirementInfo={'linktype_rmi_doors' '0000a52a (/E-STEER Core/SubSystem Specifications/Application Functions/SF009A Thermal Duty Cycle Protection)' '#SF009A_248' 'true' 'REQ: SF009A_248' '' } %GIDa_6bfff763_5252_416d_8f89_5339dea1c82a  Value=AbsltTThermLimCnt
  Constant2 : Constant  RequirementInfo={'linktype_rmi_doors' '0000a52a (/E-STEER Core/SubSystem Specifications/Application Functions/SF009A Thermal Duty Cycle Protection)' '#SF009A_148' 'true' 'REQ: SF009A_148' '' } %GIDa_659c8e78_cb9c_4371_9902_d7ea1b6ac131  Value=DutyCycThermProtnAbsltTTqSlewHiLim
  Constant3 : Constant  RequirementInfo={'linktype_rmi_doors' '0000a52a (/E-STEER Core/SubSystem Specifications/Application Functions/SF009A Thermal Duty Cycle Protection)' '#SF009A_148' 'true' 'REQ: SF009A_148' '' } %GIDa_bc6c1524_250f_48f2_9c0a_011c4c10532d  Value=DutyCycThermProtnAbsltTTqSlewLoLim
  Constant4 : Constant  RequirementInfo={'linktype_rmi_doors' '0000a52a (/E-STEER Core/SubSystem Specifications/Application Functions/SF009A Thermal Duty Cycle Protection)' '#SF009A_248' 'true' 'REQ: SF009A_248' '' } %GIDa_4fbcf33f_8768_4136_aa72_3e7081553715  Value=0
  CopyRight2 : Subsystem  Description=|  mask(Copyright Information){none=on}
      | Copyright info block.                                               
      |                                                                     
      | Place copyright information at the top of every subsystem in design.
      mask prompts: none "No parameters"
      mask help: Place copyright information at the top of every subsystem in design.
      mask Display:
      | NxtrConf = 'Nexteer Confidential';
      | 
      | sys = bdroot; %handle for the current model ("system")
      | first = get_param(sys,'Created');
      | first = first(end-3:end);  %year is last four digits
      | 
      | last = get_param(sys,'LastModifiedDate');
      | if isempty(last)
      |     last = datestr(now,'yyyy');
      | else
      |     last = last(end-3:end);
      | end
      | 
      | if strcmp(first,last)
      |     fprintf('%s -- Copyright %s Nexteer',NxtrConf,first)
      | else
      |     fprintf('%s -- %s%s- %s Nexteer',NxtrConf,char(169),first,last)
      | end
  Data Store Write1 : DataStoreWrite  DataStoreName=dDutyCycThermProtnAbsltCtrlrTTqLim
  Data Store Write2 : DataStoreWrite  DataStoreName=dDutyCycThermProtnAbsltCuTTqLim
  Data Store Write3 : DataStoreWrite  DataStoreName=dDutyCycThermProtnAbsltTTqLim
  FixdToFloat_f32_u1 : FixdToFloat/FixdToFloat_f32_u16  Param1=7
  FixdToFloat_f32_u16 : FixdToFloat/FixdToFloat_f32_u16  Param1=7
  FloatToFixd_s16_f1 : FloatToFixd/FloatToFixd_s16_f32  Param1=0
  FloatToFixd_s16_f32 : FloatToFixd/FloatToFixd_s16_f32  Param1=0
  If4 : If  RequirementInfo={'linktype_rmi_doors' '0000a52a (/E-STEER Core/SubSystem Specifications/Application Functions/SF009A Thermal Duty Cycle Protection)' '#SF009A_248' 'true' 'REQ: SF009A_248' '' } %GIDa_9d2c0776_e769_4649_a8af_b20562aa4cb7  NumInputs=2  IfExpression=u1 & u2  ElseIfExpressions=u2, u1
  Lookup Table : Lookup  RequirementInfo={'linktype_rmi_doors' '0000a52a (/E-STEER Core/SubSystem Specifications/Application Functions/SF009A Thermal Duty Cycle Protection)' '#SF009A_249' 'true' 'REQ: SF009A_249' '' ; 'linktype_rmi_doors' '0000a52a (/E-STEER Core/SubSystem Specifications/Application Functions/SF009A Thermal Duty Cycle Protection)' '#SF009A_250' 'true' 'REQ: SF009A_250' '' } %GIDa_c39bea35_9ef1_4471_9a51_0953289c9bc4  InputValues=DutyCycThermProtnAbsltCtrlTTblX  Table=DutyCycThermProtnAbsltCtrlTTqTblY  LookUpMeth=Interpolation-Use End Values  OutDataTypeStr=Inherit: Inherit via back propagation
      settings: AttributesFormatString=%<Table>\n%<InputValues>
  Lookup Table1 : Lookup  RequirementInfo={'linktype_rmi_doors' '0000a52a (/E-STEER Core/SubSystem Specifications/Application Functions/SF009A Thermal Duty Cycle Protection)' '#SF009A_251' 'true' 'REQ: SF009A_251' '' ; 'linktype_rmi_doors' '0000a52a (/E-STEER Core/SubSystem Specifications/Application Functions/SF009A Thermal Duty Cycle Protection)' '#SF009A_252' 'true' 'REQ: SF009A_252' '' } %GIDa_6c7c2055_e1a9_4038_b3df_bdcf5f63ca75  InputValues=DutyCycThermProtnAbsltCuTTblX  Table=DutyCycThermProtnAbsltCuTTqTblY  LookUpMeth=Interpolation-Use End Values  OutDataTypeStr=Inherit: Inherit via back propagation
      settings: AttributesFormatString=%<Table>\n%<InputValues>
  Merge2 : Merge  RequirementInfo={'linktype_rmi_doors' '0000a52a (/E-STEER Core/SubSystem Specifications/Application Functions/SF009A Thermal Duty Cycle Protection)' '#SF009A_248' 'true' 'REQ: SF009A_248' '' } %GIDa_f9989aea_1360_4f14_99fc_479f4d68d64e  Inputs=4
  Merge3 : Merge  RequirementInfo={'linktype_rmi_doors' '0000a52a (/E-STEER Core/SubSystem Specifications/Application Functions/SF009A Thermal Duty Cycle Protection)' '#SF009A_248' 'true' 'REQ: SF009A_248' '' } %GIDa_36886f99_bd53_4f64_b737_a87272ac1ccd  Inputs=4
  Min_f32 : NxtrMin/Min_f32  RequirementInfo={'linktype_rmi_doors' '0000a52a (/E-STEER Core/SubSystem Specifications/Application Functions/SF009A Thermal Duty Cycle Protection)' '#SF009A_147' 'true' 'REQ: SF009A_147' '' } %GIDa_e4bc48fd_2220_4af4_9908_18ec2f463133  SFunctionSpec=single y1 = Min_f32(single u1, single u2)
      settings: AttributesFormatString=%<Name>
  RateLimDyn_f32 : NxtrLim/RateLimDyn_f32  RequirementInfo={'linktype_rmi_doors' '0000a52a (/E-STEER Core/SubSystem Specifications/Application Functions/SF009A Thermal Duty Cycle Protection)' '#SF009A_148' 'true' 'REQ: SF009A_148' '' } %GIDa_5b7e70fb_4b9f_4431_8c7a_32d1bba8983c  StVar=AbsltTLimSlewStVari  Ts=ARCHGLBPRM_100MILLISEC_SEC_F32
      settings: AttributesFormatString=StVar: %<StVar>
  Relational Operator1 : RelationalOperator  RequirementInfo={'linktype_rmi_doors' '0000a52a (/E-STEER Core/SubSystem Specifications/Application Functions/SF009A Thermal Duty Cycle Protection)' '#SF009A_248' 'true' 'REQ: SF009A_248' '' } %GIDa_f72a4fcd_afc8_45e6_b80b_112afe69c19b  OutDataTypeStr=boolean
  Relational Operator4 : RelationalOperator  RequirementInfo={'linktype_rmi_doors' '0000a52a (/E-STEER Core/SubSystem Specifications/Application Functions/SF009A Thermal Duty Cycle Protection)' '#SF009A_248' 'true' 'REQ: SF009A_248' '' } %GIDa_8463a720_c548_4924_a086_e4fce8006fda  OutDataTypeStr=boolean
  Selector2 : Selector  RequirementInfo={'linktype_rmi_doors' '0000a52a (/E-STEER Core/SubSystem Specifications/Application Functions/SF009A Thermal Duty Cycle Protection)' '#SF009A_248' 'true' 'REQ: SF009A_248' '' } %GIDa_3cd35103_11e3_4e2e_9571_e27ca8d3d033  IndexMode=Zero-based  InputPortWidth=4  IndexOptions=Index vector (port)  Indices=[1 3]  OutputSizes=1
  Selector3 : Selector  RequirementInfo={'linktype_rmi_doors' '0000a52a (/E-STEER Core/SubSystem Specifications/Application Functions/SF009A Thermal Duty Cycle Protection)' '#SF009A_248' 'true' 'REQ: SF009A_248' '' } %GIDa_2dbe3dcf_f62d_449c_97c6_061994dce8a5  IndexMode=Zero-based  InputPortWidth=4  IndexOptions=Index vector (port)  Indices=[1 3]  OutputSizes=1
  SetCtrlrAndCuTFltNtc : Subsystem  RequirementInfo={'linktype_rmi_doors' '0000a52a (/E-STEER Core/SubSystem Specifications/Application Functions/SF009A Thermal Duty Cycle Protection)' '#SF009A_248' 'true' 'REQ: SF009A_248' '' } %GIDa_91afd3c0_d52f_425a_adb4_3bd6283453b3
  SetCtrlrTFltNtc : Subsystem  RequirementInfo={'linktype_rmi_doors' '0000a52a (/E-STEER Core/SubSystem Specifications/Application Functions/SF009A Thermal Duty Cycle Protection)' '#SF009A_248' 'true' 'REQ: SF009A_248' '' } %GIDa_9ea289db_5887_48a8_993d_4db16992e2cf
  SetCuTFltNtc : Subsystem  RequirementInfo={'linktype_rmi_doors' '0000a52a (/E-STEER Core/SubSystem Specifications/Application Functions/SF009A Thermal Duty Cycle Protection)' '#SF009A_248' 'true' 'REQ: SF009A_248' '' } %GIDa_19efba61_d20b_41b9_9275_ea22776d06b5
  SetNtc : Subsystem  RequirementInfo={'linktype_rmi_doors' '0000a52a (/E-STEER Core/SubSystem Specifications/Application Functions/SF009A Thermal Duty Cycle Protection)' '#SF009A_248' 'true' 'REQ: SF009A_248' '' } %GIDa_19274413_77fd_4ddd_9818_77bdf0a5393c  mask(SetNTC){}
      mask help: SetNTC library block
  SetPassdNtc : Subsystem  RequirementInfo={'linktype_rmi_doors' '0000a52a (/E-STEER Core/SubSystem Specifications/Application Functions/SF009A Thermal Duty Cycle Protection)' '#SF009A_248' 'true' 'REQ: SF009A_248' '' } %GIDa_c6d0dc5c_f478_48bb_be50_41ae6a4812a4
  Unary Minus : UnaryMinus  RequirementInfo={'linktype_rmi_doors' '0000a52a (/E-STEER Core/SubSystem Specifications/Application Functions/SF009A Thermal Duty Cycle Protection)' '#SF009A_148' 'true' 'REQ: SF009A_148' '' } %GIDa_bd6926a4_1a9f_4f10_8dae_2f4eb951abe0
  const2 : Constant  RequirementInfo={'linktype_rmi_doors' '0000a52a (/E-STEER Core/SubSystem Specifications/Application Functions/SF009A Thermal Duty Cycle Protection)' '#SF009A_248' 'true' 'REQ: SF009A_248' '' } %GIDa_fe8b26fd_766a_4c9d_9c38_b618288c4cfa  Value=DutyCycThermProtnAbsltCuTTblX
  const4 : Constant  RequirementInfo={'linktype_rmi_doors' '0000a52a (/E-STEER Core/SubSystem Specifications/Application Functions/SF009A Thermal Duty Cycle Protection)' '#SF009A_248' 'true' 'REQ: SF009A_248' '' } %GIDa_dfaebaf1_5983_4fa2_b10c_4ab2ea686540  Value=DutyCycThermProtnAbsltCtrlTTblX
  AbsTempLimitSlew : Outport
  wires:
  EcuTFild/1 -> FloatToFixd_s16_f32/1
  Lookup Table/1 -> FixdToFloat_f32_u16/1
  Min_f32/1 -> Data Store Write3/1, RateLimDyn_f32/1
  Lookup Table1/1 -> FixdToFloat_f32_u1/1
  MotWidgT/1 -> FloatToFixd_s16_f1/1
  RateLimDyn_f32/1 -> AbsTempLimitSlew/1
  Constant2/1 -> RateLimDyn_f32/3
  Constant3/1 -> Unary Minus/1
  Unary Minus/1 -> RateLimDyn_f32/2
  FloatToFixd_s16_f32/1 -> Lookup Table/1, [CtrlrTemp]
  FloatToFixd_s16_f1/1 -> Lookup Table1/1, [CuTemp]
  FixdToFloat_f32_u16/1 -> Data Store Write1/1, Min_f32/1
  FixdToFloat_f32_u1/1 -> Data Store Write2/1, Min_f32/2
  Selector2/1 -> Relational Operator1/2
  [CtrlrTemp] -> Relational Operator1/1
  [CuTemp] -> Relational Operator4/1
  const4/1 -> Selector2/1
  Constant1/1 -> Selector2/2
  const2/1 -> Selector3/1
  Constant4/1 -> Selector3/2
  Selector3/1 -> Relational Operator4/2
  Constant11/1 -> SetNtc/1(NtcNr)
  If4/1 -> SetCtrlrAndCuTFltNtc/Action
  Calibration7/1 -> SetNtc/4(DebStep)
  If4/2 -> SetCuTFltNtc/Action
  If4/3 -> SetCtrlrTFltNtc/Action
  If4/4 -> SetPassdNtc/Action
  SetCtrlrAndCuTFltNtc/1(Out1) -> Merge2/1
  SetCuTFltNtc/1(Out1) -> Merge2/2
  SetCtrlrTFltNtc/1(Out1) -> Merge2/3
  SetPassdNtc/1(Out1) -> Merge2/4
  SetPassdNtc/2(Out2) -> Merge3/4
  SetCtrlrTFltNtc/2(Out2) -> Merge3/3
  SetCuTFltNtc/2(Out2) -> Merge3/2
  SetCtrlrAndCuTFltNtc/2(Out2) -> Merge3/1
  Merge2/1 -> SetNtc/2(NtcStInfo)
  Merge3/1 -> SetNtc/3(NtcSts)
  Relational Operator4/1 -> If4/2
  Relational Operator1/1 -> If4/1
